simulink model "lipm1"  (R2023b)
settings: Solver=ode4  StartTime=0.0  StopTime=t_stop  RelTol=1e-3
values from neighbouring files (symbols this model uses):
  tao_x = 0    [data_file.m]    (also in graph_zmp.m = ans(5,:); mf2_zmp.m = u(1))
  tao_y = 0    [data_file.m]    (also in graph_zmp.m = ans(9,:); mf3_zmp.m = u(1))
  zc = 1.54    [data.m]    (also in data_file.m = 0.154; graph_file.m = ans(4,:); graph_zmp.m = ans(10,:))
settings Model: Creator=Vedang  LastModifiedBy=Vedang
settings SolverCC: AlgebraicLoopSolver=TrustRegion
settings RTWCC: DLArmComputeVersion=19.05

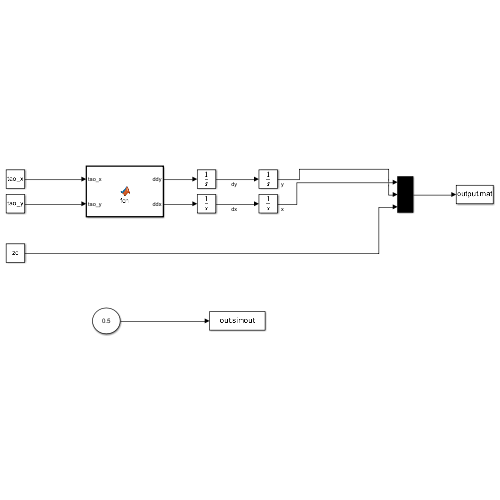
[thumbnail: Simulink's stored preview of the top-level diagram]
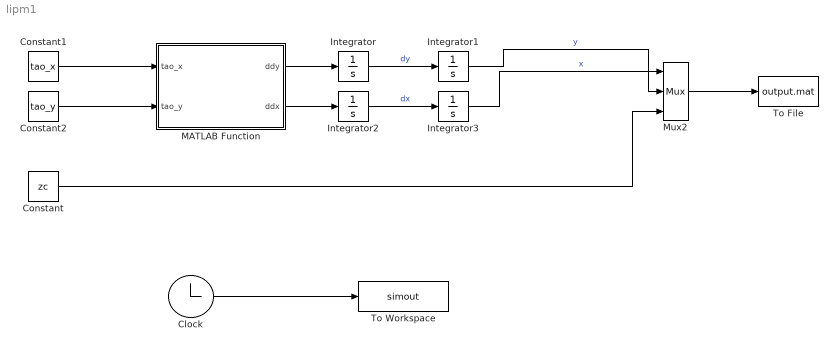
== system lipm1 ==
  Clock : Clock
  Constant : Constant  Value=zc
  Constant1 : Constant  Value=tao_x
  Constant2 : Constant  Value=tao_y
  Integrator{,1..3} (4 alike) : Integrator
  MATLAB Function : MATLAB Function  TreatAsAtomicUnit=on
  Mux2 : Mux  Inputs=3
  To File : ToFile  Filename=output.mat
  To Workspace : ToWorkspace  VariableName=simout  SaveFormat=Timeseries  SampleTime=-1
  wires:
  MATLAB Function/1(ddy) -> Integrator/1
  Integrator/1 -> Integrator1/1  "dy"
  MATLAB Function/2(ddx) -> Integrator2/1
  Integrator2/1 -> Integrator3/1  "dx"
  Integrator1/1 -> Mux2/2  "y"
  Integrator3/1 -> Mux2/1  "x"
  Constant1/1 -> MATLAB Function/1(tao_x)
  Constant2/1 -> MATLAB Function/2(tao_y)
  Mux2/1 -> To File/1
  Clock/1 -> To Workspace/1
  Constant/1 -> Mux2/3

== matlab function lipm1/MATLAB Function ==
  data: tao_x input; ddy output; tao_y input; ddx output
function [ddy,ddx] = fcn(tao_x,tao_y)
g=9.8;
zc=0.154;     %154 cm
m=58;       %58 kg
x=1;
y=2;
ddy= ((g/zc)*y - (1/(m*zc))*tao_x);
ddx= ((g/zc)*x +(1/(m*zc))*tao_y);
end
